simulink model "admire_complete_trim"  (Simulink 3.00)
settings: Solver=ode5  SolverMode=SingleTasking  StartTime=0.0  StopTime=60  FixedStep=0.02  RelTol=1e-3  AbsTol=1e-6
undefined symbols (not defined in the file or in its folder): dalpha_err, dalt_err, dbeta_err, dCl_beta, dCl_dai, dCl_day, dCl_dr, dCl_p, dCl_r, dCm_alpha, dCm_dei, dCm_dey, dCm_dne, dCm_q, dCn_beta, dCn_dna, dCn_dr, dCn_p, dCn_r, dCn_zero, dIxx, dIxz, dIyy, dIzz, dmass, dVt_err, dxcg, dycg, dzcg, u0corr, x00unc
libraries: simulink3 x22, simulink_extras x5
(part 1 of 2)
settings Model: Refine=4  SaveState=on  RTWOptions="-aLogVarNameModifier=\"rt_\" -aExtMode=0 -aRollThreshold=5 -aShowEliminatedStatements=1 -aRTWVerbose=1 -aInlineInvariantSignals=1 -aLocalBlockOutputs=1 -aInlineParameters=0"  RTWTemplateMakefile=grt_adm5p3.tmf  LastModifiedBy=lkh  ModifiedComment=nnt -- Mon Jun 05 13:08:11 2000 -- Version 3.42
settings Model: ModifiedHistory=|
  | nnt -- Mon Jun 05 13:08:11 2000 -- Version 3.42
  | 
  | 
  | nnt -- Mon Jun 05 11:01:33 2000 -- Version 3.41
  | 
  | 
  | nnt -- Mon Jun 05 10:57:40 2000 -- Version 3.40
  | 
  | 
  | nnt -- Mon Jun 05 10:56:46 2000 -- Version 3.39
  | 
  | 
  | hkg -- Thu Apr 13 16:38:30 2000 -- Version 3.38
  | Bug fix: all rate limiters were set with the canard parameters, now they get individual settings..
  | 
  | hkg -- Thu Apr 13 10:24:31 2000 -- Version 3.37
  | Inserted 3.0 version number in Level 1, changed month to April.
  | 
  | hkg -- Tue Apr 11 10:36:55 2000 -- Version 3.36
  | dtz re-connected
  | 
  | hkg -- Tue Apr 11 10:28:52 2000 -- Version 3.35
  | Changed the roll force saturation to +-80 N
  | 
  | hkg -- Tue Apr 11 09:23:02 2000 -- Version 3.34
  | All signal generators on Level 1 are now set to sine wave
  | 
  | hkg -- Mon Apr 10 15:03:16 2000 -- Version 3.33
  | New names for the RL_choice blocks
  | 
  | fosimadmin -- Mon Apr 10 13:44:14 2000 -- Version 3.32
  | Hkg actually. Nothing special
  | 
  | hkg -- Fri Apr 07 14:32:16 2000 -- Version 3.31
  | A few corrections to the names
  | 
  | hkg -- Fri Apr 07 14:16:55 2000 -- Version 3.30
  | Added unique names inside Saab and DASA rate limiters for left elevons, rudder and
  | leading-edge flaps.
  | hkg -- Fri Apr 07 14:04:35 2000 -- Version 3.29
  | Added unique names inside SAAB and DASA rate limiters for canard and right outer and
  | inner elevons.
  | hkg -- Thu Apr 06 17:23:24 2000 -- Version 3.28
  | Inserted unique names for rate limiters and multiport switches in the rate limiter selection blocks.
  | hkg -- Thu Apr 06 16:09:22 2000 -- Version 3.27
  | Disconnected dtz again. Chosen grt_adm5p3.tmf as template makefile. Code generation seems to work.
  | hyd -- Tue Mar 28 15:20:39 2000 -- Version 3.26
  | hyd -- Tue Mar 28 14:28:32 2000 -- Version 3.25
  | hyd -- Tue Mar 28 11:30:24 2000 -- Version 3.24
  | hyd -- Mon Mar 27 15:22:27 2000 -- Version 3.23
  | hyd -- Mon Mar 27 13:42:12 2000 -- Version 3.22
  | hyd -- Mon Mar 27 10:51:54 2000 -- Version 3.21
  | hyd -- Fri Mar 24 13:18:05 2000 -- Version 3.20
  | hyd -- Fri Mar 24 12:50:02 2000 -- Version 3.19
  | hyd -- Fri Mar 24 11:54:23 2000 -- Version 3.18
  | hyd -- Thu Mar 23 15:20:42 2000 -- Version 3.17
  | hyd -- Thu Mar 23 15:17:54 2000 -- Version 3.16
  | hyd -- Wed Mar 22 09:38:49 2000 -- Version 3.15
  | hyd -- Tue Mar 21 14:06:08 2000 -- Version 3.14
  | hyd -- Mon Mar 20 14:42:54 2000 -- Version 3.13
  | hyd -- Wed Mar 15 13:37:48 2000 -- Version 3.12
  | hyd -- Wed Mar 15 12:35:54 2000 -- Version 3.11
  | jnr -- Tue Mar 14 16:36:26 2000 -- Version 3.10
  | jnr -- Tue Mar 14 14:13:39 2000 -- Version 3.9
  | jnr -- Tue Mar 14 14:13:23 2000 -- Version 3.8
  | jnr -- Tue Mar 14 10:09:15 2000 -- Version 3.7
  | jnr -- Tue Mar 14 09:37:34 2000 -- Version 3.6
  | jnr -- Tue Mar 14 09:30:20 2000 -- Version 3.5
  | Add:
  | *proper stick gradients.
  | *correct gains for nz-control according to Åke Hydén.
  | *what transition region between q-control and nz-control is proper??
  | fll -- Fri Mar 03 09:53:48 2000 -- Version 3.4
  | changed name of "dtx" to "dty" (horizontal nozzle deflection)
  | fll -- Thu Mar 02 12:51:23 2000 -- Version 3.3
  | Reducesed the number of integrators to one in the longitudinal controller.
  | fll -- Thu Mar 02 12:30:52 2000 -- Version 3.2
  | Moved the blending function in the Nz and q controller.
  | fll -- Thu Mar 02 10:50:25 2000 -- Version 3.1
  | Changed input blocks to "Signal generator"
  | fll -- Thu Mar 02 10:50:25 2000 -- Version 3.0
  | Version 3.0 is modified according to comments from users

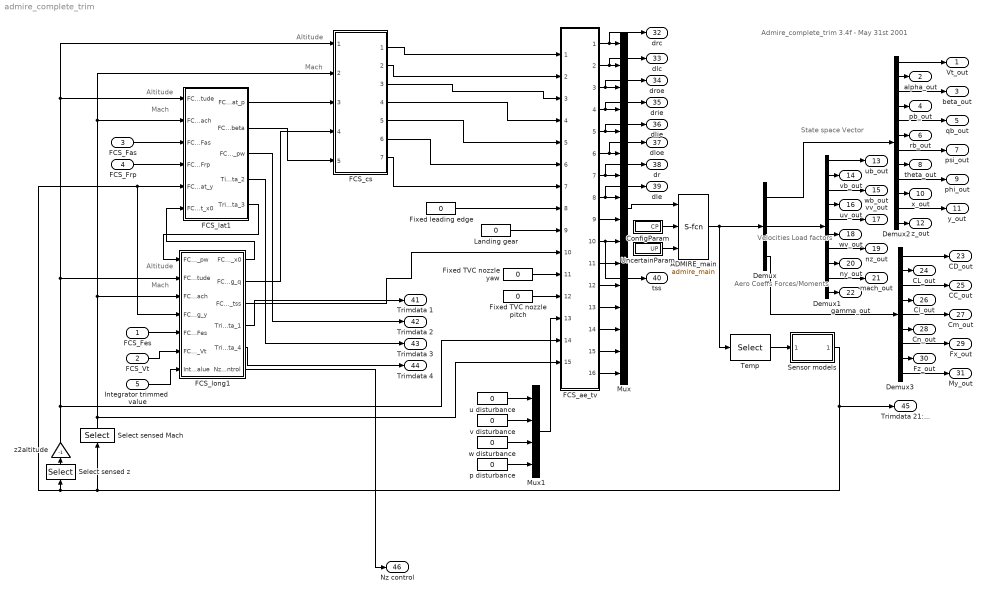
== system admire_complete_trim ==
  note: Admire_complete_trim 3.4f - May 31st 2001
  note: State space Vector
  note: Velocities
      | Load factors
  note: Aero Coeffs
      | Forces/Moments
  note: Altitude
  note: Mach
  note: Mach
  note: Altitude
  note: Altitude
  note: Mach
  FCS_Fes : Inport  Port=1  PortWidth=-1  SampleTime=-1  DataType=auto
      settings: SignalType=auto
  FCS_Vt : Inport  Port=2  PortWidth=-1  SampleTime=-1  DataType=auto
      settings: SignalType=auto
  FCS_Fas : Inport  Port=3  PortWidth=-1  SampleTime=-1  DataType=auto
      settings: SignalType=auto
  FCS_Frp : Inport  Port=4  PortWidth=-1  SampleTime=-1  DataType=auto
      settings: SignalType=auto
  Integrator trimmed  value : Inport  Port=5  PortWidth=-1  SampleTime=-1  DataType=auto
      settings: SignalType=auto
  ADMIRE_main : S-Function  FunctionName=admire_main  Parameters=x0bare zeros(12,1)  PortCounts=[]  SFunctionModules=''
      mask Type: ADMIRE C-code block
      mask Description:
      | Main block describing the ADMIRE.
      | To use HELP, start any Internet browser.
      mask Help:
      | The aircraft it self is a C-code file that calculates the dynamics of the structure and the air surrounding it.<br>
      | The simulation requires an initial vector of values called x0 containing the following variables.<br><br>
      | 
      | Vt_init     --     initial airspeed.                        [m/s]<br>
      | alpha_init --    initial angle of attack.             [rad]<br>
      | beta_init    --   initial angle of sideslip.            [rad]<br>
      | pb_init     --     initial roll angular rate.             [rad/s]<br>
      | qb_init     --     initial pitch angular rate.          [rad/s]<br>
      | rb_init       --    initial yaw angular rate.           [rad/s]<br>
      | psi_init      --    initial euler angles (azimuth)    [rad]<br>
      | theta_init   --   initial (elevation)                      [rad]<br>
      | phi_init      --   initial (bank)                             [rad]<br>
      | xv_init      --    initial x position in Fv                [m]<br>
      | yv_init        --  initial y                                     [m]<br>
      | zv_init       --   initial z                                     [m]<br>
      mask Display:
      | plot([18 12 3 2 2 8 11],[7 4 1 1 2 8 11])
      | plot([13 11 13 15 15 13],[12 11 16 17 13 12])
      | plot([15 17 20 23 30 17],[13 14 24 25 20 14])
      | plot([30 38 40 38 30],[19 31 32 22 19])
      | plot([38.5 41 36 22 41 43 36],[23 21 16 10 8 10 16])
      | plot([15 19 25 24 15],[7 9 9 8 7])
      | plot([8 11 13 14 9 8],[8 11 12 10 7 8])
      | plot([21 23],[9 10])
      | plot([30 31],[20 20.5])
  ConfigParam : Subsystem
  Demux : Demux  Outputs=[12 10 9]
  Demux1 : Demux  Outputs=10
  Demux2 : Demux  Outputs=12
  Demux3 : Demux  Outputs=9
  FCS_ae_tv : Subsystem
      mask Display: disp('Adding\ntrim\nvalues')
  "FCS_cs " : Subsystem
      mask Display: disp('FCS_cs')
  FCS_lat1 : Subsystem
      mask Display: disp('FCS_lat')
  FCS_long1 : Subsystem
      mask Display: disp('FCS_long')
  Fixed TVC nozzle pitch : Constant  Value=0
  Fixed TVC nozzle yaw : Constant  Value=0
  Fixed leading edge : Constant  Value=0
  Landing gear : Constant  Value=0
  Mux : Mux  Inputs=16
      settings: DisplayOption=none
  Mux1 : Mux  Inputs=4
      settings: DisplayOption=none
  Select sensed Mach : Selector  Orientation=up  Elements=21  InputPortWidth=28
  Select sensed z : Selector  Orientation=up  Elements=12  InputPortWidth=28
  Sensor models : Subsystem
      mask Display: disp('Sensors')
  Temp : Selector  Elements=[1:28]  InputPortWidth=31
  UncertainParam : Subsystem
      mask Display: plot([0 10 5 0],[0 0 8.6603 0])
  p disturbance : Constant  Value=0
  u disturbance : Constant  Value=0
  v disturbance : Constant  Value=0
  w disturbance : Constant  Value=0
  z2altitude : Gain  Orientation=up  Gain=-1  SaturateOnIntegerOverflow=off
  Vt_out : Outport  Port=1
  alpha_out : Outport  Port=2
  beta_out : Outport  Port=3
  pb_out : Outport  Port=4
  qb_out : Outport  Port=5
  rb_out : Outport  Port=6
  psi_out : Outport  Port=7
  theta_out : Outport  Port=8
  phi_out : Outport  Port=9
  x_out : Outport  Port=10
  y_out : Outport  Port=11
  z_out : Outport  Port=12
  ub_out : Outport  Port=13
  vb_out : Outport  Port=14
  wb_out : Outport  Port=15
  uv_out : Outport  Port=16
  vv_out : Outport  Port=17
  wv_out : Outport  Port=18
  nz_out : Outport  Port=19
  ny_out : Outport  Port=20
  mach_out : Outport  Port=21
  gamma_out : Outport  Port=22
  CD_out : Outport  Port=23
  CL_out : Outport  Port=24
  CC_out : Outport  Port=25
  Cl_out : Outport  Port=26
  Cm_out : Outport  Port=27
  Cn_out : Outport  Port=28
  Fx_out : Outport  Port=29
  Fz_out : Outport  Port=30
  My_out : Outport  Port=31
  drc : Outport  Port=32
  dlc : Outport  Port=33
  droe : Outport  Port=34
  drie : Outport  Port=35
  dlie : Outport  Port=36
  dloe : Outport  Port=37
  dr : Outport  Port=38
  dle : Outport  Port=39
  tss : Outport  Port=40
  Trimdata 1 : Outport  Port=41
  Trimdata 2 : Outport  Port=42
  Trimdata 3 : Outport  Port=43
  Trimdata 4 : Outport  Port=44
  Trimdata 21:... : Outport  Port=45
  Nz control : Outport  Port=46
  wires:
  FCS_Fes/1 -> FCS_long1/5(FCS_long_Fes)
  FCS_Vt/1 -> FCS_long1/6("FCS_long_Vt ")
  FCS_Fas/1 -> FCS_lat1/3(FCS_lat_Fas)
  FCS_Frp/1 -> FCS_lat1/4(FCS_lat_Frp)
  FCS_lat1/1("FCS_lat_p ") -> "FCS_cs "/3(FCS_cs_p)
  FCS_lat1/2("FCS_lat_beta ") -> "FCS_cs "/5(FCS_cs_beta)
  FCS_lat1/5(Trimdata_3) -> FCS_long1/1("FCS_long_pw ")
  FCS_long1/2(FCS_long_q) -> "FCS_cs "/4(FCS_cs_q)
  FCS_long1/4(Trimdata_1) -> Trimdata 1/1
  FCS_long1/5(Trimdata_4) -> Trimdata 4/1
  FCS_lat1/3(FCS_lat_pw) -> Trimdata 2/1
  FCS_lat1/4(Timdata_2) -> Trimdata 3/1
  FCS_long1/1(FCS_long_x0) -> FCS_lat1/6(FCS_lat_x0)
  Demux/1 -> Demux2/1
  Demux/3 -> Demux3/1
  ADMIRE_main/1 -> Demux/1, Temp/1
  Temp/1 -> Sensor models/1(admire_out)
  Demux3/2 -> CL_out/1
  Demux3/4 -> Cl_out/1
  Demux3/6 -> Cn_out/1
  Demux3/8 -> Fz_out/1
  Demux3/1 -> CD_out/1
  Demux3/3 -> CC_out/1
  Demux3/5 -> Cm_out/1
  Demux3/7 -> Fx_out/1
  Demux3/9 -> My_out/1
  Demux2/2 -> alpha_out/1
  Demux2/4 -> pb_out/1
  Demux2/6 -> rb_out/1
  Demux2/8 -> theta_out/1
  Demux2/10 -> x_out/1
  Demux2/12 -> z_out/1
  Demux2/1 -> Vt_out/1
  Demux2/3 -> beta_out/1
  Demux2/5 -> qb_out/1
  Demux2/7 -> psi_out/1
  Demux2/9 -> phi_out/1
  Demux2/11 -> y_out/1
  Demux/2 -> Demux1/1
  Demux1/2 -> vb_out/1
  Demux1/4 -> uv_out/1
  Demux1/6 -> wv_out/1
  Demux1/8 -> ny_out/1
  Demux1/10 -> gamma_out/1
  Demux1/1 -> ub_out/1
  Demux1/3 -> wb_out/1
  Demux1/5 -> vv_out/1
  Demux1/7 -> nz_out/1
  Demux1/9 -> mach_out/1
  ConfigParam/1(CP) -> ADMIRE_main/2
  UncertainParam/1(UP) -> ADMIRE_main/3
  Mux/1 -> ADMIRE_main/1
  FCS_ae_tv/11(FCS_ae_tv_dty_out) -> Mux/11
  FCS_ae_tv/12("FCS_ae_tv_dtz_out ") -> Mux/12
  FCS_ae_tv/13("FCS_ae_tv_u_dist_out ") -> Mux/13
  FCS_ae_tv/14("FCS_ae_tv_v_dist_out ") -> Mux/14
  FCS_ae_tv/15(FCS_ae_tv_w_dist _out) -> Mux/15
  FCS_ae_tv/16("FCS_ae_tv_p_dist_out ") -> Mux/16
  Fixed TVC nozzle pitch/1 -> FCS_ae_tv/12(FCS_ae_tv_dtz)
  Fixed TVC nozzle yaw/1 -> FCS_ae_tv/11(FCS_ae_tv_dty)
  Landing gear/1 -> FCS_ae_tv/9(FCS_ae_tv_ldg)
  Sensor models/1(admire_sensed_out) -> Trimdata 21:.../1, Select sensed z/1, FCS_long1/4(FCS_long_y), FCS_lat1/5("FCS_lat_y "), Select sensed Mach/1
  "FCS_cs "/1(FCS_cs_drc) -> FCS_ae_tv/1(FCS_ae_tv_drc)
  FCS_ae_tv/1("FCS_ae_tv_drc_out ") -> Mux/1, drc/1
  "FCS_cs "/2(FCS_cs_dlc) -> FCS_ae_tv/2(FCS_ae_tv_dlc)
  FCS_ae_tv/2("FCS_ae_tv_dlc_out ") -> Mux/2, dlc/1
  "FCS_cs "/3(FCS_cs_droe) -> FCS_ae_tv/3(FCS_ae_tv_droe)
  FCS_ae_tv/3("FCS_ae_tv_droe_out ") -> Mux/3, droe/1
  "FCS_cs "/4(FCS_cs_drie) -> FCS_ae_tv/4(FCS_ae_tv_drie)
  FCS_ae_tv/4("FCS_ae_tv_drie_out ") -> Mux/4, drie/1
  "FCS_cs "/5(FCS_cs_dlie) -> FCS_ae_tv/5(FCS_ae_tv_dlie)
  FCS_ae_tv/5("FCS_ae_tv_dlie_out ") -> Mux/5, dlie/1
  "FCS_cs "/6(FCS_cs_dloe) -> FCS_ae_tv/6(FCS_ae_tv_dloe)
  FCS_ae_tv/6("FCS_ae_tv_dloe_out ") -> Mux/6, dloe/1
  "FCS_cs "/7(FCS_cs_dr) -> FCS_ae_tv/7(FCS_ae_tv_dr)
  FCS_ae_tv/7(FCS_ae_tv_dr _out) -> Mux/7, dr/1
  Fixed leading edge/1 -> FCS_ae_tv/8(FCS_ae_tv_dle)
  FCS_ae_tv/8("FCS_ae_tv_dle_out ") -> Mux/8, dle/1
  FCS_long1/3(FCS_long_tss) -> FCS_ae_tv/10(FCS_ae_tv_tss)
  FCS_ae_tv/9(FCS_ae_tv_ldg_out) -> Mux/9
  FCS_ae_tv/10("FCS_ae_tv_tss_out ") -> Mux/10, tss/1
  Integrator trimmed  value/1 -> FCS_long1/7(Integrator value)
  Mux1/1 -> FCS_ae_tv/13(FCS_ae_tv_dist)
  p disturbance/1 -> Mux1/4
  w disturbance/1 -> Mux1/3
  v disturbance/1 -> Mux1/2
  u disturbance/1 -> Mux1/1
  Select sensed z/1 -> z2altitude/1
  Select sensed Mach/1 -> FCS_long1/3(FCS_long_Mach), "FCS_cs "/2(FCS_cs_Mach), FCS_lat1/2("FCS_lat_Mach "), FCS_ae_tv/15(Mach)
  z2altitude/1 -> FCS_long1/2("FCS_long_Altitude "), FCS_lat1/1("FCS_lat_Altitude "), "FCS_cs "/1(FCS_cs_Altitude), FCS_ae_tv/14(Altitude)
  FCS_long1/6(Nz control) -> Nz control/1

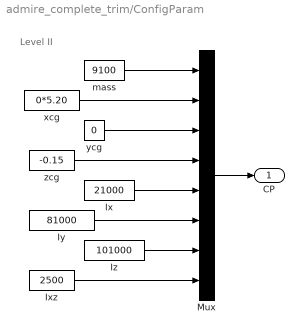
== system admire_complete_trim/ConfigParam ==
  note: Level II
  "Ix " : Constant  Value=21000
  "Ixz " : Constant  Value=2500
  "Iy " : Constant  Value=81000
  "Iz " : Constant  Value=101000
  Mux : Mux  Inputs=8
      settings: DisplayOption=none
  "mass " : Constant  Value=9100
  "xcg " : Constant  Value=0*5.20
  "ycg " : Constant  Value=0
  "zcg " : Constant  Value=-0.15
  CP : Outport  Port=1  InitialOutput=0
  wires:
  "mass "/1 -> Mux/1
  "xcg "/1 -> Mux/2
  "ycg "/1 -> Mux/3
  "zcg "/1 -> Mux/4
  "Ix "/1 -> Mux/5
  "Iy "/1 -> Mux/6
  "Iz "/1 -> Mux/7
  "Ixz "/1 -> Mux/8
  Mux/1 -> CP/1

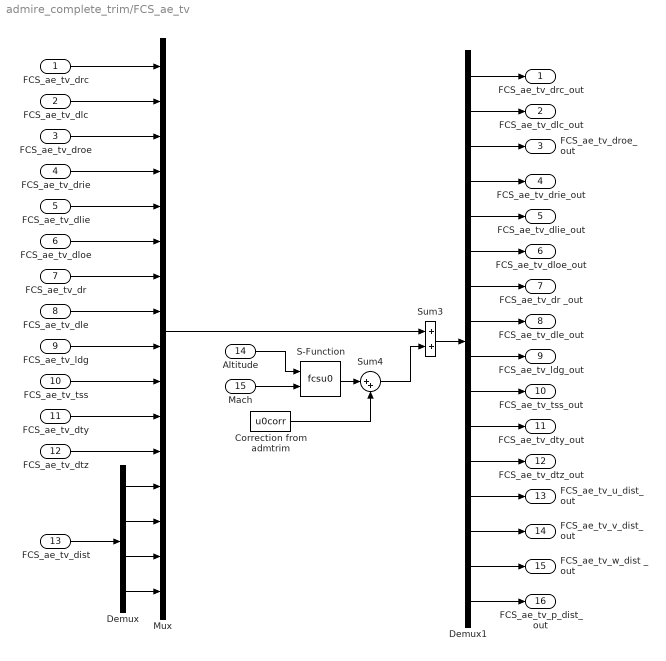
== system admire_complete_trim/FCS_ae_tv ==
  FCS_ae_tv_drc : Inport  Port=1  PortWidth=-1  SampleTime=-1  DataType=auto
      settings: SignalType=auto
  FCS_ae_tv_dlc : Inport  Port=2  PortWidth=-1  SampleTime=-1  DataType=auto
      settings: SignalType=auto
  FCS_ae_tv_droe : Inport  Port=3  PortWidth=-1  SampleTime=-1  DataType=auto
      settings: SignalType=auto
  FCS_ae_tv_drie : Inport  Port=4  PortWidth=-1  SampleTime=-1  DataType=auto
      settings: SignalType=auto
  FCS_ae_tv_dlie : Inport  Port=5  PortWidth=-1  SampleTime=-1  DataType=auto
      settings: SignalType=auto
  FCS_ae_tv_dloe : Inport  Port=6  PortWidth=-1  SampleTime=-1  DataType=auto
      settings: SignalType=auto
  FCS_ae_tv_dr : Inport  Port=7  PortWidth=-1  SampleTime=-1  DataType=auto
      settings: SignalType=auto
  FCS_ae_tv_dle : Inport  Port=8  PortWidth=-1  SampleTime=-1  DataType=auto
      settings: SignalType=auto
  FCS_ae_tv_ldg : Inport  Port=9  PortWidth=-1  SampleTime=-1  DataType=auto
      settings: SignalType=auto
  FCS_ae_tv_tss : Inport  Port=10  PortWidth=-1  SampleTime=-1  DataType=auto
      settings: SignalType=auto
  FCS_ae_tv_dty : Inport  Port=11  PortWidth=-1  SampleTime=-1  DataType=auto
      settings: SignalType=auto
  FCS_ae_tv_dtz : Inport  Port=12  PortWidth=-1  SampleTime=-1  DataType=auto
      settings: SignalType=auto
  FCS_ae_tv_dist : Inport  Port=13  PortWidth=-1  SampleTime=-1  DataType=auto
      settings: SignalType=auto
  Altitude : Inport  Port=14  PortWidth=-1  SampleTime=-1  DataType=auto
      settings: SignalType=auto
  Mach : Inport  Port=15  PortWidth=-1  SampleTime=-1  DataType=auto
      settings: SignalType=auto
  Correction from admtrim : Constant  Value=u0corr
  Demux : Demux  Outputs=4
  Demux1 : Demux  Outputs=16
  Mux : Mux  Inputs=16
  S-Function : S-Function  FunctionName=fcsu0  PortCounts=[]  SFunctionModules=''
  Sum3 : Sum  Inputs=++  SaturateOnIntegerOverflow=on
  Sum4 : Sum  Inputs=|++  SaturateOnIntegerOverflow=on
  "FCS_ae_tv_drc_out " : Outport  Port=1
  "FCS_ae_tv_dlc_out " : Outport  Port=2
  "FCS_ae_tv_droe_out " : Outport  Port=3
  "FCS_ae_tv_drie_out " : Outport  Port=4
  "FCS_ae_tv_dlie_out " : Outport  Port=5
  "FCS_ae_tv_dloe_out " : Outport  Port=6
  FCS_ae_tv_dr _out : Outport  Port=7
  "FCS_ae_tv_dle_out " : Outport  Port=8
  FCS_ae_tv_ldg_out : Outport  Port=9
  "FCS_ae_tv_tss_out " : Outport  Port=10
  FCS_ae_tv_dty_out : Outport  Port=11
  "FCS_ae_tv_dtz_out " : Outport  Port=12
  "FCS_ae_tv_u_dist_out " : Outport  Port=13
  "FCS_ae_tv_v_dist_out " : Outport  Port=14
  FCS_ae_tv_w_dist _out : Outport  Port=15
  "FCS_ae_tv_p_dist_out " : Outport  Port=16
  wires:
  FCS_ae_tv_dist/1 -> Demux/1
  FCS_ae_tv_drc/1 -> Mux/1
  FCS_ae_tv_dlc/1 -> Mux/2
  FCS_ae_tv_droe/1 -> Mux/3
  FCS_ae_tv_drie/1 -> Mux/4
  FCS_ae_tv_dlie/1 -> Mux/5
  FCS_ae_tv_dloe/1 -> Mux/6
  FCS_ae_tv_dr/1 -> Mux/7
  FCS_ae_tv_dle/1 -> Mux/8
  FCS_ae_tv_dty/1 -> Mux/11
  FCS_ae_tv_dtz/1 -> Mux/12
  Demux/1 -> Mux/13
  Demux/2 -> Mux/14
  Demux/3 -> Mux/15
  Demux/4 -> Mux/16
  FCS_ae_tv_ldg/1 -> Mux/9
  FCS_ae_tv_tss/1 -> Mux/10
  Sum3/1 -> Demux1/1
  Demux1/3 -> "FCS_ae_tv_droe_out "/1
  Demux1/4 -> "FCS_ae_tv_drie_out "/1
  Demux1/5 -> "FCS_ae_tv_dlie_out "/1
  Demux1/6 -> "FCS_ae_tv_dloe_out "/1
  Demux1/7 -> FCS_ae_tv_dr _out/1
  Demux1/8 -> "FCS_ae_tv_dle_out "/1
  Demux1/11 -> FCS_ae_tv_dty_out/1
  Demux1/12 -> "FCS_ae_tv_dtz_out "/1
  Demux1/13 -> "FCS_ae_tv_u_dist_out "/1
  Demux1/14 -> "FCS_ae_tv_v_dist_out "/1
  Demux1/15 -> FCS_ae_tv_w_dist _out/1
  Demux1/16 -> "FCS_ae_tv_p_dist_out "/1
  Demux1/2 -> "FCS_ae_tv_dlc_out "/1
  Demux1/1 -> "FCS_ae_tv_drc_out "/1
  Mux/1 -> Sum3/1
  S-Function/1 -> Sum4/1
  Correction from admtrim/1 -> Sum4/2
  Demux1/9 -> FCS_ae_tv_ldg_out/1
  Demux1/10 -> "FCS_ae_tv_tss_out "/1
  Altitude/1 -> S-Function/1
  Mach/1 -> S-Function/2
  Sum4/1 -> Sum3/2

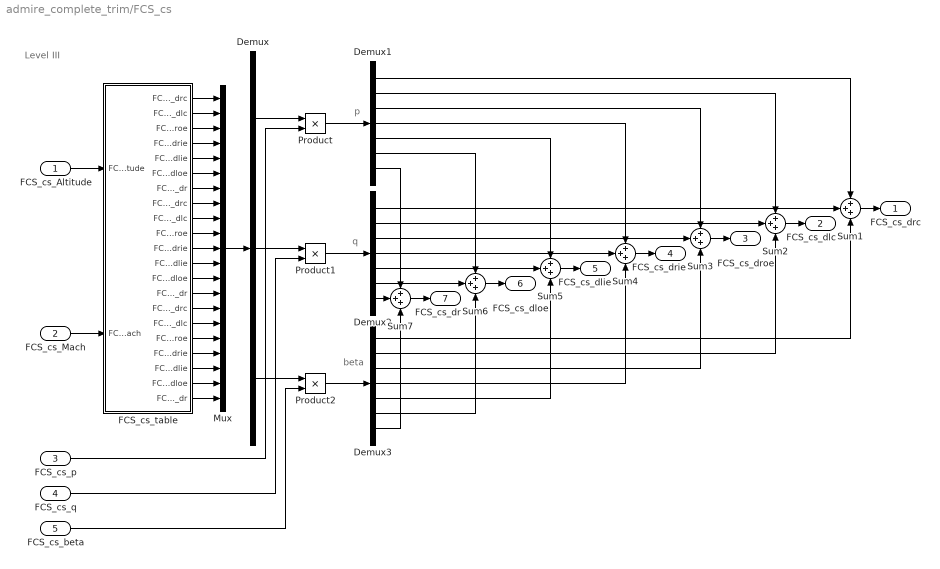
== system admire_complete_trim/FCS_cs  ==
  note: Level III
  note: beta
  note: q
  note: p
  FCS_cs_Altitude : Inport  Port=1  PortWidth=-1  SampleTime=-1  DataType=auto
      settings: SignalType=auto
  FCS_cs_Mach : Inport  Port=2  PortWidth=-1  SampleTime=-1  DataType=auto
      settings: SignalType=auto
  FCS_cs_p : Inport  Port=3  PortWidth=-1  SampleTime=-1  DataType=auto
      settings: SignalType=auto
  FCS_cs_q : Inport  Port=4  PortWidth=-1  SampleTime=-1  DataType=auto
      settings: SignalType=auto
  FCS_cs_beta : Inport  Port=5  PortWidth=-1  SampleTime=-1  DataType=auto
      settings: SignalType=auto
  Demux : Demux  Outputs=[7 7 7]
  Demux1 : Demux  Outputs=7
  Demux2 : Demux  Outputs=7
  Demux3 : Demux  Outputs=7
  FCS_cs_table : Subsystem
      mask Display: disp('FCS_cs_table')
  Mux : Mux  Inputs=21
  Product : Product  Inputs=2  SaturateOnIntegerOverflow=on
  Product1 : Product  Inputs=2  SaturateOnIntegerOverflow=on
  Product2 : Product  Inputs=2  SaturateOnIntegerOverflow=on
  Sum{1..7} (7 alike) : Sum  Inputs=3  SaturateOnIntegerOverflow=on
  FCS_cs_drc : Outport  Port=1
  FCS_cs_dlc : Outport  Port=2
  FCS_cs_droe : Outport  Port=3
  FCS_cs_drie : Outport  Port=4
  FCS_cs_dlie : Outport  Port=5
  FCS_cs_dloe : Outport  Port=6
  FCS_cs_dr : Outport  Port=7
  wires:
  Sum1/1 -> FCS_cs_drc/1
  Demux3/1 -> Sum1/3
  Demux1/1 -> Sum1/1
  Sum2/1 -> FCS_cs_dlc/1
  Demux3/2 -> Sum2/3
  Demux1/2 -> Sum2/1
  Demux2/1 -> Sum1/2
  Sum3/1 -> FCS_cs_droe/1
  Demux3/3 -> Sum3/3
  Demux1/3 -> Sum3/1
  Demux2/2 -> Sum2/2
  Sum4/1 -> FCS_cs_drie/1
  Demux3/4 -> Sum4/3
  Demux1/4 -> Sum4/1
  Demux2/3 -> Sum3/2
  Sum5/1 -> FCS_cs_dlie/1
  Demux3/5 -> Sum5/3
  Demux1/5 -> Sum5/1
  Demux2/4 -> Sum4/2
  Sum6/1 -> FCS_cs_dloe/1
  Demux3/6 -> Sum6/3
  Demux1/6 -> Sum6/1
  Demux2/5 -> Sum5/2
  Sum7/1 -> FCS_cs_dr/1
  Demux3/7 -> Sum7/3
  Demux1/7 -> Sum7/1
  Demux2/7 -> Sum7/2
  Demux2/6 -> Sum6/2
  Product2/1 -> Demux3/1
  Product1/1 -> Demux2/1
  Product/1 -> Demux1/1
  FCS_cs_table/21(FCS_cs_table_beta_dr) -> Mux/21
  FCS_cs_table/20(FCS_cs_table_beta_dloe) -> Mux/20
  FCS_cs_table/19(FCS_cs_table_beta_dlie) -> Mux/19
  FCS_cs_table/18(FCS_cs_table_beta_drie) -> Mux/18
  FCS_cs_table/17(FCS_cs_table_beta_droe) -> Mux/17
  FCS_cs_table/16(FCS_cs_table_beta_dlc) -> Mux/16
  FCS_cs_table/15(FCS_cs_table_beta_drc) -> Mux/15
  FCS_cs_table/13(FCS_cs_table_q_dloe) -> Mux/13
  FCS_cs_table/14(FCS_cs_table_q_dr) -> Mux/14
  FCS_cs_table/12(FCS_cs_table_q_dlie) -> Mux/12
  FCS_cs_table/11(FCS_cs_table_q_drie) -> Mux/11
  FCS_cs_table/10(FCS_cs_table_q_droe) -> Mux/10
  FCS_cs_table/9(FCS_cs_table_q_dlc) -> Mux/9
  FCS_cs_table/8(FCS_cs_table_q_drc) -> Mux/8
  FCS_cs_table/7(FCS_cs_table_p_dr) -> Mux/7
  FCS_cs_table/6(FCS_cs_table_p_dloe) -> Mux/6
  FCS_cs_table/5(FCS_cs_table_p_dlie) -> Mux/5
  FCS_cs_table/4(FCS_cs_table_p_drie) -> Mux/4
  FCS_cs_table/3(FCS_cs_table_p_droe) -> Mux/3
  FCS_cs_table/2(FCS_cs_table_p_dlc) -> Mux/2
  FCS_cs_table/1(FCS_cs_table_p_drc) -> Mux/1
  FCS_cs_Mach/1 -> FCS_cs_table/2(FCS_cs_table_Mach)
  FCS_cs_Altitude/1 -> FCS_cs_table/1(FCS_cs_table_Altitude)
  FCS_cs_beta/1 -> Product2/2
  FCS_cs_q/1 -> Product1/2
  FCS_cs_p/1 -> Product/2
  Demux/3 -> Product2/1
  Demux/2 -> Product1/1
  Demux/1 -> Product/1
  Mux/1 -> Demux/1

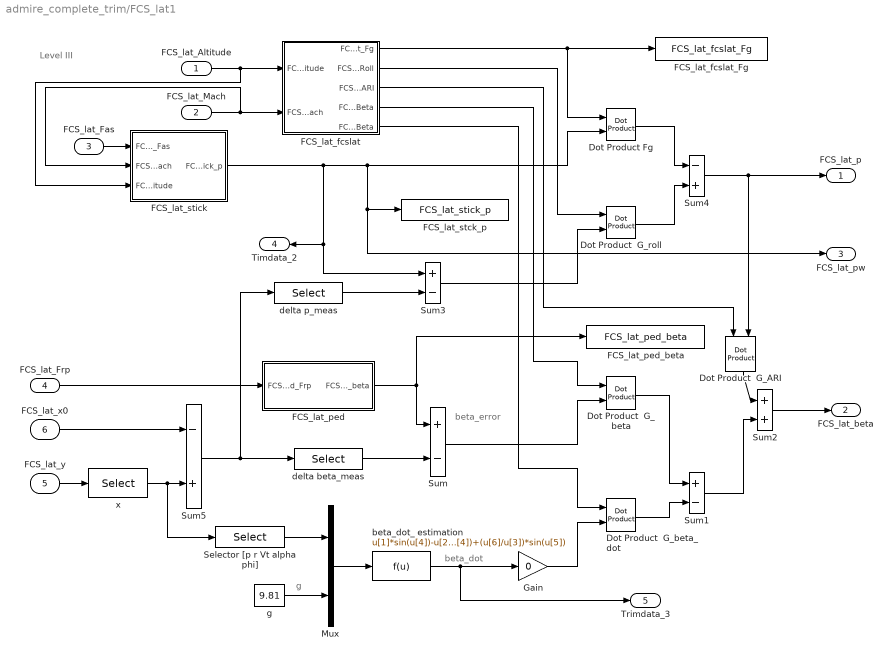
== system admire_complete_trim/FCS_lat1 ==
  note: g
  note: beta_dot
  note: beta_error
  note: Level III
  "FCS_lat_Altitude " : Inport  Port=1  PortWidth=-1  SampleTime=-1  DataType=auto
      settings: SignalType=auto
  "FCS_lat_Mach " : Inport  Port=2  PortWidth=-1  SampleTime=-1  DataType=auto
      settings: SignalType=auto
  FCS_lat_Fas : Inport  Port=3  PortWidth=-1  SampleTime=-1  DataType=auto
      settings: SignalType=auto
  FCS_lat_Frp : Inport  Port=4  PortWidth=-1  SampleTime=-1  DataType=auto
      settings: SignalType=auto
  "FCS_lat_y " : Inport  Port=5  PortWidth=-1  SampleTime=-1  DataType=auto
      settings: SignalType=auto
  FCS_lat_x0 : Inport  Port=6  PortWidth=-1  SampleTime=-1  DataType=auto
      settings: SignalType=auto
  "  x" : Selector  Elements=[1:12]  InputPortWidth=28
  Dot Product Fg : simulink3/Math/Dot Product
  Dot Product  G_ARI : simulink3/Math/Dot Product  Orientation=down
  Dot Product  G_beta : simulink3/Math/Dot Product
  Dot Product  G_beta_dot : simulink3/Math/Dot Product
  Dot Product  G_roll : simulink3/Math/Dot Product
  FCS_lat_fcslat : Subsystem
      mask Display: disp('Calc of lateral\namplfication\n factors')
  FCS_lat_fcslat_Fg : ToWorkspace  VariableName=FCS_lat_fcslat_Fg  SampleTime=-1  SaveFormat=Matrix
  FCS_lat_ped : Subsystem
      mask Display: disp('FCS lateral pedal\nforce N to beta rad')
  FCS_lat_ped_beta : ToWorkspace  VariableName=FCS_lat_ped_beta  SampleTime=-1  SaveFormat=Matrix
  FCS_lat_stck_p : ToWorkspace  VariableName=FCS_lat_stick_p  SampleTime=-1  SaveFormat=Matrix
  FCS_lat_stick : Subsystem
      mask Display: disp('FCS lateral stick\ngradient\n N to rad/s')
  Gain : Gain  Gain=0  SaturateOnIntegerOverflow=on
  Mux : Mux  Inputs=2
      settings: DisplayOption=none
  Selector [p r Vt alpha phi] : Selector  Elements=[4 6 1 2 9]  InputPortWidth=12
  Sum : Sum  Inputs=+-  SaturateOnIntegerOverflow=on
  Sum1 : Sum  Inputs=+-  SaturateOnIntegerOverflow=on
  Sum2 : Sum  Inputs=++  SaturateOnIntegerOverflow=on
  Sum3 : Sum  Inputs=+-  SaturateOnIntegerOverflow=on
  Sum4 : Sum  Inputs=-+  SaturateOnIntegerOverflow=on
  Sum5 : Sum  Inputs=-+  SaturateOnIntegerOverflow=on
  beta_dot_ estimation : Fcn  Expr=u[1]*sin(u[4])-u[2]*cos(u[4])+(u[6]/u[3])*sin(u[5])
  delta beta_meas : Selector  Elements=3  InputPortWidth=12
  delta p_meas : Selector  Elements=4  InputPortWidth=12
  g : Constant  Value=9.81
  "FCS_lat_p " : Outport  Port=1  InitialOutput=0
  "FCS_lat_beta " : Outport  Port=2  InitialOutput=0
  FCS_lat_pw : Outport  Port=3  InitialOutput=0
  Timdata_2 : Outport  Orientation=left  Port=4  InitialOutput=0
  Trimdata_3 : Outport  Port=5  InitialOutput=0
  wires:
  FCS_lat_Fas/1 -> FCS_lat_stick/1("FCS_lat_stick_Fas ")
  delta p_meas/1 -> Sum3/2
  Mux/1 -> beta_dot_ estimation/1
  Selector [p r Vt alpha phi]/1 -> Mux/1
  g/1 -> Mux/2
  Sum3/1 -> Dot Product  G_roll/2
  Dot Product  G_roll/1 -> Sum4/2
  Dot Product Fg/1 -> Sum4/1
  Dot Product  G_beta/1 -> Sum1/1
  Dot Product  G_beta_dot/1 -> Sum1/2
  Sum4/1 -> Dot Product  G_ARI/2, "FCS_lat_p "/1
  Dot Product  G_ARI/1 -> Sum2/1
  Sum2/1 -> "FCS_lat_beta "/1
  Sum1/1 -> Sum2/2
  FCS_lat_stick/1(FCS_lat_stick_p) -> Dot Product Fg/2, FCS_lat_pw/1, FCS_lat_stck_p/1, Sum3/1, Timdata_2/1
  FCS_lat_fcslat/2(FCS_lat_fcslat_GRoll) -> Dot Product  G_roll/1
  FCS_lat_fcslat/3(FCS_lat_fcslat_GARI) -> Dot Product  G_ARI/1
  FCS_lat_fcslat/4(FCS_lat_fcslat_GBeta) -> Dot Product  G_beta/1
  FCS_lat_fcslat/5(FCS_lat_fcslat_dGBeta) -> Dot Product  G_beta_dot/1
  delta beta_meas/1 -> Sum/2
  Sum/1 -> Dot Product  G_beta/2
  FCS_lat_Frp/1 -> FCS_lat_ped/1(FCS_lat_ped_Frp)
  FCS_lat_ped/1(FCS_lat_ped_beta) -> Sum/1, FCS_lat_ped_beta/1
  "FCS_lat_Altitude "/1 -> FCS_lat_fcslat/1(FCS_lat_fcslat_Altitude), FCS_lat_stick/3("FCS_lat_stick_Altitude ")
  "FCS_lat_Mach "/1 -> FCS_lat_stick/2("FCS_lat_stick_Mach "), FCS_lat_fcslat/2(FCS_lat_fcslat_Mach)
  "FCS_lat_y "/1 -> "  x"/1
  FCS_lat_x0/1 -> Sum5/1
  "  x"/1 -> Sum5/2, Selector [p r Vt alpha phi]/1
  Sum5/1 -> delta beta_meas/1, delta p_meas/1
  FCS_lat_fcslat/1(FCS_lat_fcslat_Fg) -> Dot Product Fg/1, FCS_lat_fcslat_Fg/1
  Gain/1 -> Dot Product  G_beta_dot/2
  beta_dot_ estimation/1 -> Gain/1, Trimdata_3/1

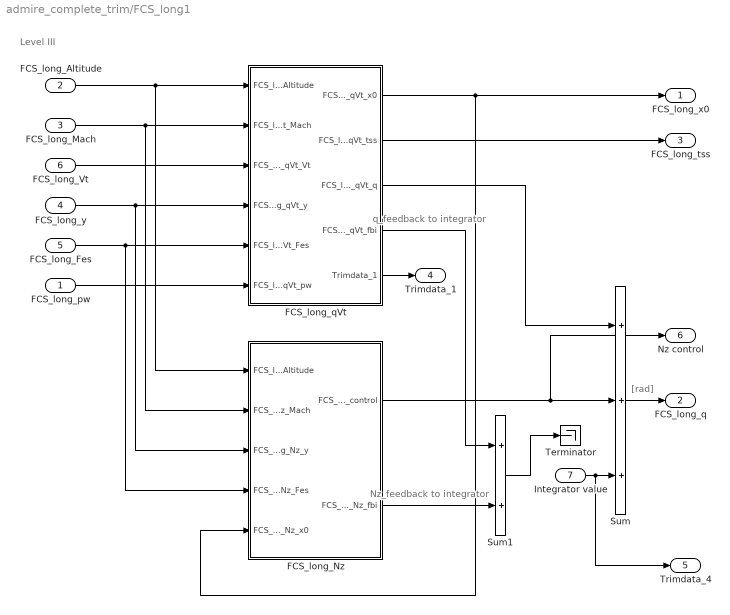
== system admire_complete_trim/FCS_long1 ==
  note: Level III
  note: q_feedback
      | to integrator
  note: Nz_feedback
      | to integrator
  note: [rad]
  "FCS_long_pw " : Inport  Port=1  PortWidth=-1  SampleTime=-1  DataType=auto
      settings: SignalType=auto
  "FCS_long_Altitude " : Inport  Port=2  PortWidth=-1  SampleTime=-1  DataType=auto
      settings: SignalType=auto
  FCS_long_Mach : Inport  Port=3  PortWidth=-1  SampleTime=-1  DataType=auto
      settings: SignalType=auto
  FCS_long_y : Inport  Port=4  PortWidth=-1  SampleTime=-1  DataType=auto
      settings: SignalType=auto
  FCS_long_Fes : Inport  Port=5  PortWidth=-1  SampleTime=-1  DataType=auto
      settings: SignalType=auto
  "FCS_long_Vt " : Inport  Port=6  PortWidth=-1  SampleTime=-1  DataType=auto
      settings: SignalType=auto
  Integrator value : Inport  Port=7  PortWidth=-1  SampleTime=-1  DataType=auto
      settings: SignalType=auto
  FCS_long_Nz : Subsystem
      mask Display: disp('FCS_long_Nz')
  FCS_long_qVt : Subsystem
      mask Display: disp('FCS_long_qVt')
  Sum : Sum  Inputs=+++  SaturateOnIntegerOverflow=on
  Sum1 : Sum  Inputs=++  SaturateOnIntegerOverflow=on
  Terminator : Terminator
  FCS_long_x0 : Outport  Port=1  InitialOutput=0
  FCS_long_q : Outport  Port=2  InitialOutput=0
  FCS_long_tss : Outport  Port=3  InitialOutput=0
  Trimdata_1 : Outport  Port=4  InitialOutput=0
  Trimdata_4 : Outport  Port=5  InitialOutput=0
  Nz control : Outport  Port=6  InitialOutput=0
  wires:
  "FCS_long_Vt "/1 -> FCS_long_qVt/3(FCS_long_qVt_Vt)
  FCS_long_Mach/1 -> FCS_long_qVt/2(FCS_long_qVt_Mach), FCS_long_Nz/2("FCS_long_Nz_Mach ")
  FCS_long_y/1 -> FCS_long_qVt/4(FCS_long_qVt_y), FCS_long_Nz/3(FCS_long_Nz_y)
  FCS_long_qVt/1(FCS_long_qVt_x0) -> FCS_long_x0/1, FCS_long_Nz/5(FCS_long_Nz_x0)
  FCS_long_Fes/1 -> FCS_long_qVt/5(FCS_long_qVt_Fes), FCS_long_Nz/4(FCS_long_Nz_Fes)
  "FCS_long_pw "/1 -> FCS_long_qVt/6("FCS_long_qVt_pw ")
  FCS_long_qVt/2(FCS_long_qVt_tss) -> FCS_long_tss/1
  FCS_long_qVt/3(FCS_long_qVt_q) -> Sum/1
  FCS_long_qVt/4(FCS_long_qVt_fbi) -> Sum1/1
  FCS_long_Nz/2(FCS_long_Nz_fbi) -> Sum1/2
  "FCS_long_Altitude "/1 -> FCS_long_qVt/1(FCS_long_qVt_Altitude), FCS_long_Nz/1("FCS_long_Nz_Altitude ")
  Sum/1 -> FCS_long_q/1
  FCS_long_qVt/5(Trimdata_1) -> Trimdata_1/1
  Integrator value/1 -> Sum/3, Trimdata_4/1
  Sum1/1 -> Terminator/1
  FCS_long_Nz/1(FCS_long_Nz_control) -> Sum/2, Nz control/1

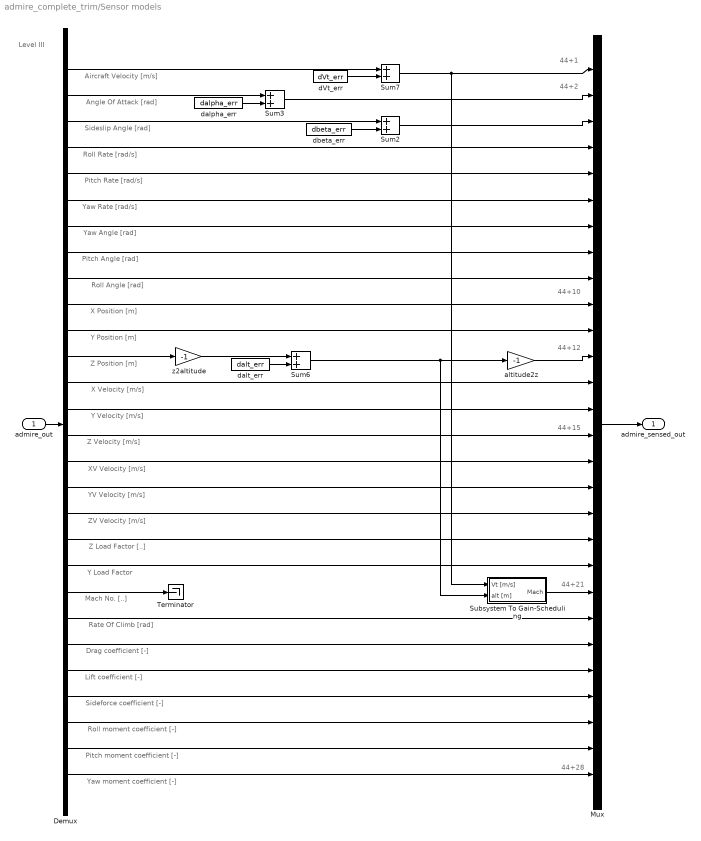
== system admire_complete_trim/Sensor models ==
  note: Aircraft Velocity [m/s]
  note: Angle Of Attack [rad]
  note: Sideslip Angle [rad]
  note: Roll Rate [rad/s]
  note: Pitch Rate [rad/s]
  note: Yaw Rate [rad/s]
  note: Yaw Angle [rad]
  note: Pitch Angle [rad]
  note: Roll Angle [rad]
  note: X Position [m]
  note: Y Position [m]
  note: Z Position [m]
  note: X Velocity [m/s]
  note: Y Velocity [m/s]
  note: Z Velocity [m/s]
  note: ZV Velocity [m/s]
  note: YV Velocity [m/s]
  note: XV Velocity [m/s]
  note: Z Load Factor [..]
  note: Y Load Factor
  note: Mach No. [..]
  note: Rate Of Climb [rad]
  note: Drag coefficient [-]
  note: Lift coefficient [-]
  note: Sideforce coefficient [-]
  note: Roll moment coefficient [-]
  note: Pitch moment coefficient [-]
  note: Yaw moment coefficient [-]
  note: Level III
  note: 44+1
  note: 44+2
  note: 44+10
  note: 44+15
  note: 44+21
  note: 44+28
  note: 44+12
  admire_out : Inport  Port=1  PortWidth=-1  SampleTime=-1  DataType=auto
      settings: SignalType=auto
  Demux : Demux  Outputs=28
  Mux : Mux  Inputs=28
      settings: DisplayOption=none
  Subsystem To Gain-Scheduling : Subsystem
  Sum{2..3,6..7} (4 alike) : Sum  Inputs=++  SaturateOnIntegerOverflow=on
  Terminator : Terminator
  altitude2z : Gain  Gain=-1  SaturateOnIntegerOverflow=off
  dVt_err : Constant  Value=dVt_err
  dalpha_err : Constant  Value=dalpha_err
  dalt_err : Constant  Value=dalt_err
  dbeta_err : Constant  Value=dbeta_err
  z2altitude : Gain  Gain=-1  SaturateOnIntegerOverflow=off
  admire_sensed_out : Outport  Port=1
  wires:
  Demux/24 -> Mux/24
  Demux/25 -> Mux/25
  Demux/26 -> Mux/26
  Demux/27 -> Mux/27
  Demux/28 -> Mux/28
  admire_out/1 -> Demux/1
  Demux/11 -> Mux/11
  Demux/13 -> Mux/13
  Demux/14 -> Mux/14
  Demux/15 -> Mux/15
  Demux/16 -> Mux/16
  Demux/17 -> Mux/17
  Demux/18 -> Mux/18
  Demux/20 -> Mux/20
  Demux/22 -> Mux/22
  Demux/23 -> Mux/23
  Demux/21 -> Terminator/1
  Mux/1 -> admire_sensed_out/1
  Subsystem To Gain-Scheduling/1(Mach) -> Mux/21
  Demux/7 -> Mux/7
  dalt_err/1 -> Sum6/2
  Demux/12 -> z2altitude/1
  z2altitude/1 -> Sum6/1
  Demux/10 -> Mux/10
  Sum7/1 -> Mux/1, Subsystem To Gain-Scheduling/1(Vt [m/s])
  Sum2/1 -> Mux/3
  Demux/4 -> Mux/4
  Demux/5 -> Mux/5
  Demux/6 -> Mux/6
  Demux/8 -> Mux/8
  Demux/9 -> Mux/9
  Demux/19 -> Mux/19
  dalpha_err/1 -> Sum3/2
  Demux/2 -> Sum3/1
  dbeta_err/1 -> Sum2/2
  Demux/3 -> Sum2/1
  Sum3/1 -> Mux/2
  dVt_err/1 -> Sum7/2
  Demux/1 -> Sum7/1
  Sum6/1 -> Subsystem To Gain-Scheduling/2(alt [m]), altitude2z/1
  altitude2z/1 -> Mux/12

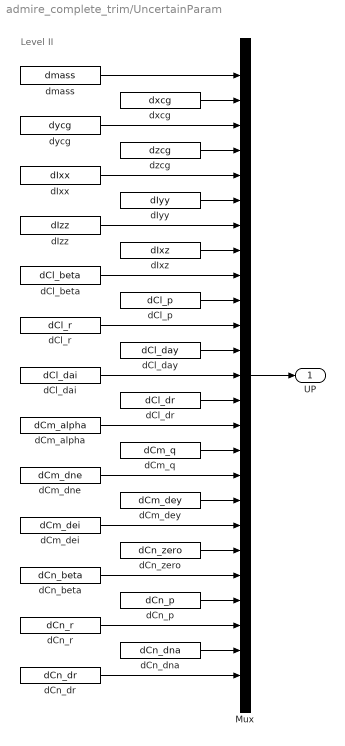
== system admire_complete_trim/UncertainParam ==
  note: Level II
  Mux : Mux  Inputs=25
      settings: DisplayOption=none
  "dCl_beta " : Constant  Value=dCl_beta
  "dCl_dai " : Constant  Value=dCl_dai
  dCl_day : Constant  Value=dCl_day
  "dCl_dr " : Constant  Value=dCl_dr
  "dCl_p " : Constant  Value=dCl_p
  "dCl_r " : Constant  Value=dCl_r
  "dCm_alpha " : Constant  Value=dCm_alpha
  "dCm_dei " : Constant  Value=dCm_dei
  "dCm_dey " : Constant  Value=dCm_dey
  "dCm_dne " : Constant  Value=dCm_dne
  "dCm_q " : Constant  Value=dCm_q
  "dCn_beta " : Constant  Value=dCn_beta
  dCn_dna : Constant  Value=dCn_dna
  "dCn_dr " : Constant  Value=dCn_dr
  "dCn_p " : Constant  Value=dCn_p
  "dCn_r " : Constant  Value=dCn_r
  dCn_zero : Constant  Value=dCn_zero
  dIxx : Constant  Value=dIxx
  dIxz : Constant  Value=dIxz
  "dIyy " : Constant  Value=dIyy
  "dIzz " : Constant  Value=dIzz
  "dmass " : Constant  Value=dmass
  dxcg : Constant  Value=dxcg
  "dycg " : Constant  Value=dycg
  "dzcg " : Constant  Value=dzcg
  UP : Outport  Port=1  InitialOutput=0
  wires:
  dCn_dna/1 -> Mux/24
  "dmass "/1 -> Mux/1
  "dycg "/1 -> Mux/3
  dxcg/1 -> Mux/2
  "dzcg "/1 -> Mux/4
  dIxx/1 -> Mux/5
  "dIyy "/1 -> Mux/6
  "dIzz "/1 -> Mux/7
  dIxz/1 -> Mux/8
  "dCl_beta "/1 -> Mux/9
  "dCl_p "/1 -> Mux/10
  "dCl_r "/1 -> Mux/11
  dCl_day/1 -> Mux/12
  "dCl_dai "/1 -> Mux/13
  "dCl_dr "/1 -> Mux/14
  "dCm_alpha "/1 -> Mux/15
  "dCm_q "/1 -> Mux/16
  "dCm_dey "/1 -> Mux/18
  dCn_zero/1 -> Mux/20
  "dCn_p "/1 -> Mux/22
  Mux/1 -> UP/1
  "dCm_dne "/1 -> Mux/17
  "dCm_dei "/1 -> Mux/19
  "dCn_beta "/1 -> Mux/21
  "dCn_dr "/1 -> Mux/25
  "dCn_r "/1 -> Mux/23

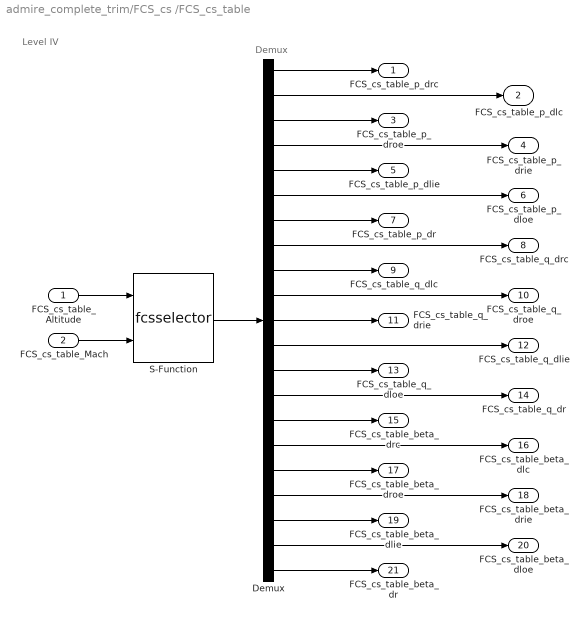
== system admire_complete_trim/FCS_cs /FCS_cs_table ==
  note: Demux
  note: Level IV
  FCS_cs_table_Altitude : Inport  Port=1  PortWidth=-1  SampleTime=-1  DataType=auto
      settings: SignalType=auto
  FCS_cs_table_Mach : Inport  Port=2  PortWidth=-1  SampleTime=-1  DataType=auto
      settings: SignalType=auto
  Demux : Demux  Outputs=21
  S-Function : S-Function  FunctionName=fcsselector  PortCounts=[]  SFunctionModules=''
  FCS_cs_table_p_drc : Outport  Port=1
  FCS_cs_table_p_dlc : Outport  Port=2
  FCS_cs_table_p_droe : Outport  Port=3
  FCS_cs_table_p_drie : Outport  Port=4
  FCS_cs_table_p_dlie : Outport  Port=5
  FCS_cs_table_p_dloe : Outport  Port=6
  FCS_cs_table_p_dr : Outport  Port=7
  FCS_cs_table_q_drc : Outport  Port=8
  FCS_cs_table_q_dlc : Outport  Port=9
  FCS_cs_table_q_droe : Outport  Port=10
  FCS_cs_table_q_drie : Outport  Port=11
  FCS_cs_table_q_dlie : Outport  Port=12
  FCS_cs_table_q_dloe : Outport  Port=13
  FCS_cs_table_q_dr : Outport  Port=14
  FCS_cs_table_beta_drc : Outport  Port=15
  FCS_cs_table_beta_dlc : Outport  Port=16
  FCS_cs_table_beta_droe : Outport  Port=17
  FCS_cs_table_beta_drie : Outport  Port=18
  FCS_cs_table_beta_dlie : Outport  Port=19
  FCS_cs_table_beta_dloe : Outport  Port=20
  FCS_cs_table_beta_dr : Outport  Port=21
  wires:
  Demux/1 -> FCS_cs_table_p_drc/1
  Demux/14 -> FCS_cs_table_q_dr/1
  Demux/20 -> FCS_cs_table_beta_dloe/1
  Demux/18 -> FCS_cs_table_beta_drie/1
  Demux/16 -> FCS_cs_table_beta_dlc/1
  Demux/12 -> FCS_cs_table_q_dlie/1
  Demux/10 -> FCS_cs_table_q_droe/1
  Demux/8 -> FCS_cs_table_q_drc/1
  Demux/6 -> FCS_cs_table_p_dloe/1
  Demux/4 -> FCS_cs_table_p_drie/1
  Demux/2 -> FCS_cs_table_p_dlc/1
  Demux/21 -> FCS_cs_table_beta_dr/1
  Demux/19 -> FCS_cs_table_beta_dlie/1
  Demux/17 -> FCS_cs_table_beta_droe/1
  Demux/15 -> FCS_cs_table_beta_drc/1
  Demux/13 -> FCS_cs_table_q_dloe/1
  Demux/11 -> FCS_cs_table_q_drie/1
  Demux/9 -> FCS_cs_table_q_dlc/1
  Demux/7 -> FCS_cs_table_p_dr/1
  Demux/5 -> FCS_cs_table_p_dlie/1
  Demux/3 -> FCS_cs_table_p_droe/1
  S-Function/1 -> Demux/1
  FCS_cs_table_Mach/1 -> S-Function/2
  FCS_cs_table_Altitude/1 -> S-Function/1

== system admire_complete_trim/FCS_lat1/FCS_lat_fcslat ==
  note: Level IV
  note: S-function
  FCS_lat_fcslat_Altitude : Inport  Port=1  PortWidth=-1  SampleTime=-1  DataType=auto
      settings: SignalType=auto
  FCS_lat_fcslat_Mach : Inport  Port=2  PortWidth=-1  SampleTime=-1  DataType=auto
      settings: SignalType=auto
  S-Function : S-Function  FunctionName=fcslateral  PortCounts=[]  SFunctionModules=''
  FCS_lat_fcslat_Fg : Outport  Port=1
  FCS_lat_fcslat_GRoll : Outport  Port=2
  FCS_lat_fcslat_GARI : Outport  Port=3
  FCS_lat_fcslat_GBeta : Outport  Port=4
  FCS_lat_fcslat_dGBeta : Outport  Port=5
  wires:
  FCS_lat_fcslat_Altitude/1 -> S-Function/1
  FCS_lat_fcslat_Mach/1 -> S-Function/2
  S-Function/1 -> FCS_lat_fcslat_Fg/1
  S-Function/2 -> FCS_lat_fcslat_GBeta/1
  S-Function/3 -> FCS_lat_fcslat_dGBeta/1
  S-Function/4 -> FCS_lat_fcslat_GARI/1
  S-Function/5 -> FCS_lat_fcslat_GRoll/1

== system admire_complete_trim/FCS_lat1/FCS_lat_ped ==
  note: Level IV
  FCS_lat_ped_Frp : Inport  Port=1  PortWidth=-1  SampleTime=-1  DataType=auto
      settings: SignalType=auto
  Degrees to Radians : simulink_extras/Transformations/Degrees to Radians
  Look-Up Table Frp gradient : Lookup  InputValues=[-200 0 200]  OutputValues=[5 0 -5]
  Saturation : Saturate  UpperLimit=200  LowerLimit=-200
  FCS_lat_ped_beta : Outport  Port=1
  wires:
  Saturation/1 -> Look-Up Table Frp gradient/1
  FCS_lat_ped_Frp/1 -> Saturation/1
  Degrees to Radians/1 -> FCS_lat_ped_beta/1
  Look-Up Table Frp gradient/1 -> Degrees to Radians/1

== system admire_complete_trim/FCS_lat1/FCS_lat_stick ==
  note: Level IV
  "FCS_lat_stick_Fas " : Inport  Port=1  PortWidth=-1  SampleTime=-1  DataType=auto
      settings: SignalType=auto
  "FCS_lat_stick_Mach " : Inport  Port=2  PortWidth=-1  SampleTime=-1  DataType=auto
      settings: SignalType=auto
  "FCS_lat_stick_Altitude " : Inport  Port=3  PortWidth=-1  SampleTime=-1  DataType=auto
      settings: SignalType=auto
  Degrees to Radians : simulink_extras/Transformations/Degrees to Radians
  Gain : Gain  Gain=180/80  SaturateOnIntegerOverflow=on
  Saturation : Saturate  UpperLimit=80  LowerLimit=-80
  Terminator : Terminator
  Terminator 2 : Terminator
  FCS_lat_stick_p : Outport  Port=1
  wires:
  "FCS_lat_stick_Fas "/1 -> Saturation/1
  Degrees to Radians/1 -> FCS_lat_stick_p/1
  Saturation/1 -> Gain/1
  Gain/1 -> Degrees to Radians/1
  "FCS_lat_stick_Mach "/1 -> Terminator/1
  "FCS_lat_stick_Altitude "/1 -> Terminator 2/1

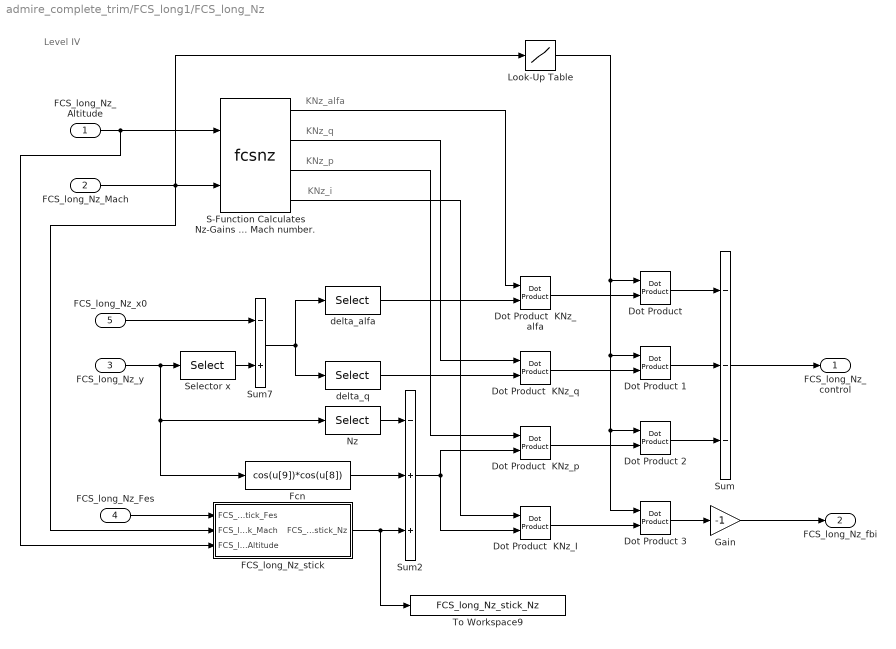
== system admire_complete_trim/FCS_long1/FCS_long_Nz ==
  note: KNz_alfa
  note: KNz_q
  note: KNz_p
  note: KNz_i
  note: Level IV
  "FCS_long_Nz_Altitude " : Inport  Port=1  PortWidth=-1  SampleTime=-1  DataType=auto
      settings: SignalType=auto
  "FCS_long_Nz_Mach " : Inport  Port=2  PortWidth=-1  SampleTime=-1  DataType=auto
      settings: SignalType=auto
  FCS_long_Nz_y : Inport  Port=3  PortWidth=-1  SampleTime=-1  DataType=auto
      settings: SignalType=auto
  FCS_long_Nz_Fes : Inport  Port=4  PortWidth=-1  SampleTime=-1  DataType=auto
      settings: SignalType=auto
  FCS_long_Nz_x0 : Inport  Port=5  PortWidth=-1  SampleTime=-1  DataType=auto
      settings: SignalType=auto
  Dot Product {,1..3} (4 alike) : simulink3/Math/Dot Product
  Dot Product  KNz_I : simulink3/Math/Dot Product
  Dot Product  KNz_alfa : simulink3/Math/Dot Product
  Dot Product  KNz_p : simulink3/Math/Dot Product
  Dot Product  KNz_q : simulink3/Math/Dot Product
  FCS_long_Nz_stick : Subsystem
      mask Display: disp('FCS_long_Nz_stick')
  Fcn : Fcn  Expr=cos(u[9])*cos(u[8])
  Gain : Gain  Gain=-1  SaturateOnIntegerOverflow=on
  Look-Up Table : Lookup  InputValues=[0 0.58 0.62 2.5]  OutputValues=[0 0 1 1]
  Nz : Selector  Elements=19  InputPortWidth=28
  S-Function Calculates Nz-Gains as a function of altitude and Mach number. : S-Function  FunctionName=fcsnz  PortCounts=[]  SFunctionModules=''
  Selector x : Selector  Elements=[1:12]  InputPortWidth=28
  Sum : Sum  Inputs=---  SaturateOnIntegerOverflow=on
  Sum2 : Sum  Inputs=-++  SaturateOnIntegerOverflow=on
  Sum7 : Sum  Inputs=-+  SaturateOnIntegerOverflow=on
  To Workspace9 : ToWorkspace  VariableName=FCS_long_Nz_stick_Nz  SampleTime=-1  SaveFormat=Matrix
  delta_alfa : Selector  Elements=2  InputPortWidth=12
  delta_q : Selector  Elements=5  InputPortWidth=12
  FCS_long_Nz_control : Outport  Port=1
  FCS_long_Nz_fbi : Outport  Port=2
  wires:
  Nz/1 -> Sum2/1
  FCS_long_Nz_Fes/1 -> FCS_long_Nz_stick/1("FCS_long_Nz_stick_Fes ")
  Selector x/1 -> Sum7/2
  FCS_long_Nz_x0/1 -> Sum7/1
  Sum7/1 -> delta_alfa/1, delta_q/1
  FCS_long_Nz_y/1 -> Selector x/1, Nz/1, Fcn/1
  "FCS_long_Nz_Mach "/1 -> S-Function Calculates Nz-Gains as a function of altitude and Mach number./2, Look-Up Table/1, FCS_long_Nz_stick/2(FCS_long_Nz_stick_Mach)
  Sum2/1 -> Dot Product  KNz_p/2, Dot Product  KNz_I/2
  S-Function Calculates Nz-Gains as a function of altitude and Mach number./4 -> Dot Product  KNz_I/1
  delta_alfa/1 -> Dot Product  KNz_alfa/2
  delta_q/1 -> Dot Product  KNz_q/2
  S-Function Calculates Nz-Gains as a function of altitude and Mach number./3 -> Dot Product  KNz_p/1
  S-Function Calculates Nz-Gains as a function of altitude and Mach number./2 -> Dot Product  KNz_q/1
  S-Function Calculates Nz-Gains as a function of altitude and Mach number./1 -> Dot Product  KNz_alfa/1
  "Dot Product "/1 -> Sum/1
  Dot Product  KNz_alfa/1 -> "Dot Product "/2
  Dot Product 1/1 -> Sum/2
  Dot Product  KNz_q/1 -> Dot Product 1/2
  Look-Up Table/1 -> "Dot Product "/1, Dot Product 1/1, Dot Product 2/1, Dot Product 3/1
  Dot Product 2/1 -> Sum/3
  Dot Product  KNz_p/1 -> Dot Product 2/2
  Dot Product  KNz_I/1 -> Dot Product 3/2
  Sum/1 -> FCS_long_Nz_control/1
  Gain/1 -> FCS_long_Nz_fbi/1
  Dot Product 3/1 -> Gain/1
  "FCS_long_Nz_Altitude "/1 -> S-Function Calculates Nz-Gains as a function of altitude and Mach number./1, FCS_long_Nz_stick/3("FCS_long_Nz_stick_Altitude ")
  FCS_long_Nz_stick/1(FCS_long_Nz_stick_Nz) -> To Workspace9/1, Sum2/3
  Fcn/1 -> Sum2/2

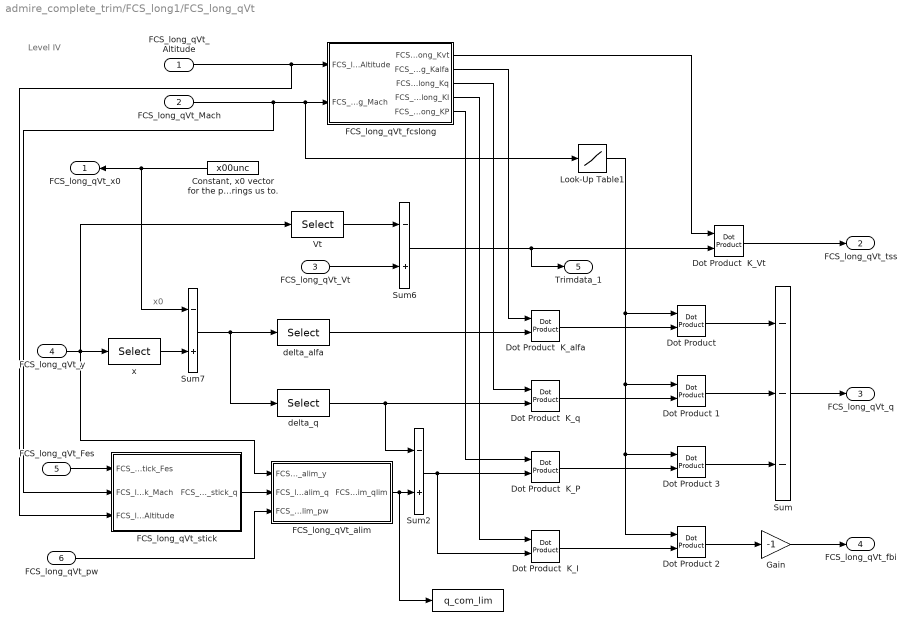
== system admire_complete_trim/FCS_long1/FCS_long_qVt ==
  note: x0
  note: Level IV
  FCS_long_qVt_Altitude : Inport  Port=1  PortWidth=-1  SampleTime=-1  DataType=auto
      settings: SignalType=auto
  FCS_long_qVt_Mach : Inport  Port=2  PortWidth=-1  SampleTime=-1  DataType=auto
      settings: SignalType=auto
  FCS_long_qVt_Vt : Inport  Port=3  PortWidth=-1  SampleTime=-1  DataType=auto
      settings: SignalType=auto
  FCS_long_qVt_y : Inport  Port=4  PortWidth=-1  SampleTime=-1  DataType=auto
      settings: SignalType=auto
  FCS_long_qVt_Fes : Inport  Port=5  PortWidth=-1  SampleTime=-1  DataType=auto
      settings: SignalType=auto
  "FCS_long_qVt_pw " : Inport  Port=6  PortWidth=-1  SampleTime=-1  DataType=auto
      settings: SignalType=auto
  " " : ToWorkspace  VariableName=q_com_lim  SampleTime=-1  SaveFormat=Matrix
  "Constant, x0 vector for the point that the sensor uncertainties  brings us to." : Constant  Orientation=left  Value=x00unc
  Dot Product {,1..3} (4 alike) : simulink3/Math/Dot Product
  Dot Product  K_I : simulink3/Math/Dot Product
  Dot Product  K_P : simulink3/Math/Dot Product
  Dot Product  K_Vt : simulink3/Math/Dot Product
  Dot Product  K_alfa : simulink3/Math/Dot Product
  Dot Product  K_q : simulink3/Math/Dot Product
  FCS_long_qVt_alim : Subsystem
      mask Display: disp('FCS_long_qVt_alim')
  FCS_long_qVt_fcslong : Subsystem
      mask Display: disp('FCS_long_qVt_fcslong')
  FCS_long_qVt_stick : Subsystem
      mask Display: disp('FCS_long_qVt_stick')
  Gain : Gain  Gain=-1  SaturateOnIntegerOverflow=on
  Look-Up Table1 : Lookup  InputValues=[0 0.58 0.62 2.5]  OutputValues=[1 1 0 0]
  Sum : Sum  Inputs=---  SaturateOnIntegerOverflow=on
  Sum2 : Sum  Inputs=-+  SaturateOnIntegerOverflow=on
  Sum6 : Sum  Inputs=-+  SaturateOnIntegerOverflow=on
  Sum7 : Sum  Inputs=-+  SaturateOnIntegerOverflow=on
  Vt : Selector  Elements=1  InputPortWidth=28
  delta_alfa : Selector  Elements=2  InputPortWidth=12
  delta_q : Selector  Elements=5  InputPortWidth=12
  x : Selector  Elements=[1:12]  InputPortWidth=28
  FCS_long_qVt_x0 : Outport  Orientation=left  Port=1
  FCS_long_qVt_tss : Outport  Port=2
  FCS_long_qVt_q : Outport  Port=3
  FCS_long_qVt_fbi : Outport  Port=4
  Trimdata_1 : Outport  Port=5
  wires:
  FCS_long_qVt_fcslong/4(FCS_long_qVt_fcslong_KI) -> Dot Product  K_I/1
  FCS_long_qVt_fcslong/5(FCS_long_qVt_fcslong_KP) -> Dot Product  K_P/1
  FCS_long_qVt_Altitude/1 -> FCS_long_qVt_fcslong/1(FCS_long_qVt_fcslong_Altitude), FCS_long_qVt_stick/3("FCS_long_qVt_stick_Altitude ")
  FCS_long_qVt_Mach/1 -> FCS_long_qVt_fcslong/2(FCS_long_qVt_fcslong_Mach), Look-Up Table1/1, FCS_long_qVt_stick/2("FCS_long_qVt_stick_Mach ")
  delta_alfa/1 -> Dot Product  K_alfa/2
  x/1 -> Sum7/2
  Sum7/1 -> delta_alfa/1, delta_q/1
  delta_q/1 -> Dot Product  K_q/2, Sum2/1
  FCS_long_qVt_y/1 -> x/1, Vt/1, FCS_long_qVt_alim/1(FCS_long_qVt_alim_y)
  FCS_long_qVt_Fes/1 -> FCS_long_qVt_stick/1("FCS_long_qVt_stick_Fes ")
  FCS_long_qVt_alim/1(FCS_long_qVt_alim_qlim) -> Sum2/2, " "/1
  FCS_long_qVt_stick/1("FCS_long_qVt_stick_q ") -> FCS_long_qVt_alim/2("FCS_long_qVt_alim_q ")
  "FCS_long_qVt_pw "/1 -> FCS_long_qVt_alim/3(FCS_long_qVt_alim_pw)
  Dot Product  K_Vt/1 -> FCS_long_qVt_tss/1
  FCS_long_qVt_fcslong/1(FCS_long_qVt_fcslong_Kvt) -> Dot Product  K_Vt/1
  Sum2/1 -> Dot Product  K_P/2, Dot Product  K_I/2
  Dot Product  K_P/1 -> Dot Product 3/2
  Dot Product  K_I/1 -> Dot Product 2/2
  Sum/1 -> FCS_long_qVt_q/1
  Dot Product  K_q/1 -> Dot Product 1/2
  Dot Product 1/1 -> Sum/2
  "Dot Product "/1 -> Sum/1
  Dot Product  K_alfa/1 -> "Dot Product "/2
  Look-Up Table1/1 -> "Dot Product "/1, Dot Product 1/1, Dot Product 2/1, Dot Product 3/1
  Dot Product 3/1 -> Sum/3
  Gain/1 -> FCS_long_qVt_fbi/1
  Dot Product 2/1 -> Gain/1
  FCS_long_qVt_fcslong/3(FCS_long_qVt_fcslong_Kq) -> Dot Product  K_q/1
  FCS_long_qVt_fcslong/2(FCS_long_qVt_fcslong_Kalfa) -> Dot Product  K_alfa/1
  FCS_long_qVt_Vt/1 -> Sum6/2
  Sum6/1 -> Dot Product  K_Vt/2, Trimdata_1/1
  Vt/1 -> Sum6/1
  "Constant, x0 vector for the point that the sensor uncertainties  brings us to."/1 -> FCS_long_qVt_x0/1, Sum7/1

== system admire_complete_trim/Sensor models/Subsystem To Gain-Scheduling ==
  note: Level III
  Vt [m/s] : Inport  Port=1  PortWidth=-1  SampleTime=-1  DataType=auto
      settings: SignalType=auto
  alt [m] : Inport  Port=2  PortWidth=-1  SampleTime=-1  DataType=auto
      settings: SignalType=auto
  S-Function : S-Function  FunctionName=machno  PortCounts=[]  SFunctionModules=''
  Mach : Outport  Port=1
  wires:
  Vt [m/s]/1 -> S-Function/1
  S-Function/1 -> Mach/1
  alt [m]/1 -> S-Function/2

== system admire_complete_trim/FCS_long1/FCS_long_Nz/FCS_long_Nz_stick ==
  note: Level V
  "FCS_long_Nz_stick_Fes " : Inport  Port=1  PortWidth=-1  SampleTime=-1  DataType=auto
      settings: SignalType=auto
  FCS_long_Nz_stick_Mach : Inport  Port=2  PortWidth=-1  SampleTime=-1  DataType=auto
      settings: SignalType=auto
  "FCS_long_Nz_stick_Altitude " : Inport  Port=3  PortWidth=-1  SampleTime=-1  DataType=auto
      settings: SignalType=auto
  Gain : Gain  Gain=8/80  SaturateOnIntegerOverflow=on
  Saturation [-40,+80]   [Newton] : Saturate  UpperLimit=80  LowerLimit=-40
  Terminator : Terminator
  Terminator 2 : Terminator
  FCS_long_Nz_stick_Nz : Outport  Port=1
  wires:
  "FCS_long_Nz_stick_Fes "/1 -> Saturation [-40,+80]   [Newton]/1
  Saturation [-40,+80]   [Newton]/1 -> Gain/1
  Gain/1 -> FCS_long_Nz_stick_Nz/1
  "FCS_long_Nz_stick_Altitude "/1 -> Terminator 2/1
  FCS_long_Nz_stick_Mach/1 -> Terminator/1

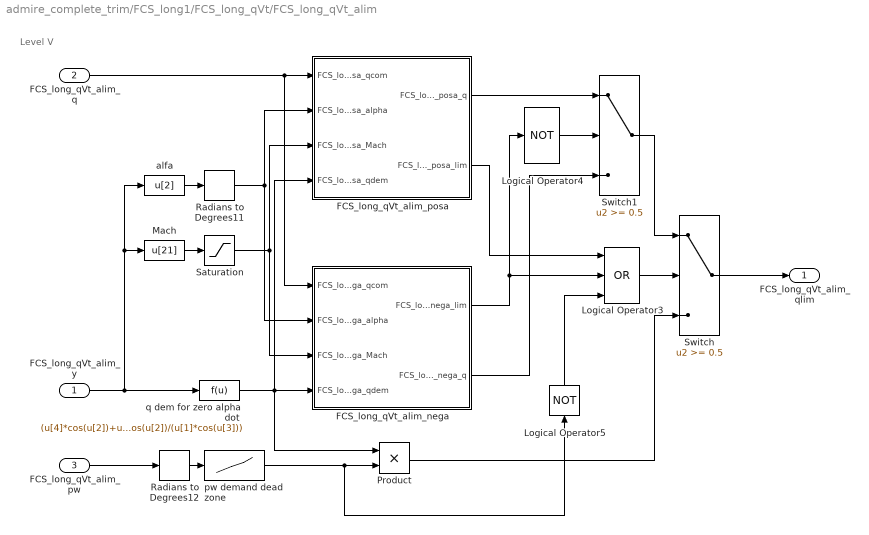
== system admire_complete_trim/FCS_long1/FCS_long_qVt/FCS_long_qVt_alim ==
  note: Level V
  FCS_long_qVt_alim_y : Inport  Port=1  PortWidth=-1  SampleTime=-1  DataType=auto
      settings: SignalType=auto
  "FCS_long_qVt_alim_q " : Inport  Port=2  PortWidth=-1  SampleTime=-1  DataType=auto
      settings: SignalType=auto
  FCS_long_qVt_alim_pw : Inport  Port=3  PortWidth=-1  SampleTime=-1  DataType=auto
      settings: SignalType=auto
  FCS_long_qVt_alim_nega : Subsystem
      mask Display: disp('FCS_long_qVt_alim\nnegative alpha')
  FCS_long_qVt_alim_posa : Subsystem
      mask Display: disp('FCS_long_qVt_alim\npositive alpha')
  Logical Operator3 : Logic  Operator=OR  Inputs=3
  Logical Operator4 : Logic  Operator=NOT  Inputs=1
  Logical Operator5 : Logic  Orientation=up  Operator=NOT  Inputs=1
  Mach : Fcn  Expr=u[21]
  Product : Product  Inputs=2  SaturateOnIntegerOverflow=on
  Radians to Degrees11 : simulink_extras/Transformations/Radians to Degrees
  Radians to Degrees12 : simulink_extras/Transformations/Radians to Degrees
  Saturation : Saturate  UpperLimit=2.5  LowerLimit=0
  Switch : Switch  Threshold=0.5
  Switch1 : Switch  Threshold=0.5
  alfa : Fcn  Expr=u[2]
  pw demand dead zone : Lookup  InputValues=[-180 -10 -8 8 10 180]  OutputValues=[0 0 0 0 0 0]
  "q dem for zero alpha dot " : Fcn  Expr=(u[4]*cos(u[2])+u[6]*sin(u[2]))*tan(u[3])+(u[19]-cos(u[8])*cos(u[9]))*9.80665*cos(u[2])/(u[1]*cos(u[3]))
  FCS_long_qVt_alim_qlim : Outport  Port=1
  wires:
  Logical Operator3/1 -> Switch/2
  Switch1/1 -> Switch/1
  alfa/1 -> Radians to Degrees11/1
  Mach/1 -> Saturation/1
  Radians to Degrees11/1 -> FCS_long_qVt_alim_posa/2("FCS_long_qVt_alim_posa_alpha "), FCS_long_qVt_alim_nega/2("FCS_long_qVt_alim_nega_alpha ")
  Saturation/1 -> FCS_long_qVt_alim_posa/3("FCS_long_qVt_alim_posa_Mach "), FCS_long_qVt_alim_nega/3("FCS_long_qVt_alim_nega_Mach ")
  FCS_long_qVt_alim_y/1 -> "q dem for zero alpha dot "/1, Mach/1, alfa/1
  "q dem for zero alpha dot "/1 -> FCS_long_qVt_alim_nega/4("FCS_long_qVt_alim_nega_qdem "), FCS_long_qVt_alim_posa/4("FCS_long_qVt_alim_posa_qdem "), Product/1
  "FCS_long_qVt_alim_q "/1 -> FCS_long_qVt_alim_posa/1("FCS_long_qVt_alim_posa_qcom "), FCS_long_qVt_alim_nega/1("FCS_long_qVt_alim_nega_qcom ")
  FCS_long_qVt_alim_nega/2("FCS_long_qVt_alim_nega_q ") -> Switch1/3
  FCS_long_qVt_alim_posa/1(FCS_long_qVt_alim_posa_q) -> Switch1/1
  Logical Operator4/1 -> Switch1/2
  FCS_long_qVt_alim_nega/1(FCS_long_qVt_alim_nega_lim) -> Logical Operator4/1, Logical Operator3/2
  FCS_long_qVt_alim_posa/2(FCS_long_qVt_alim_posa_lim) -> Logical Operator3/1
  Switch/1 -> FCS_long_qVt_alim_qlim/1
  Radians to Degrees12/1 -> pw demand dead zone/1
  Product/1 -> Switch/3
  FCS_long_qVt_alim_pw/1 -> Radians to Degrees12/1
  pw demand dead zone/1 -> Product/2, Logical Operator5/1
  Logical Operator5/1 -> Logical Operator3/3

== system admire_complete_trim/FCS_long1/FCS_long_qVt/FCS_long_qVt_fcslong ==
  note: Level V
  note: S-function
  FCS_long_qVt_fcslong_Altitude : Inport  Port=1  PortWidth=-1  SampleTime=-1  DataType=auto
      settings: SignalType=auto
  FCS_long_qVt_fcslong_Mach : Inport  Port=2  PortWidth=-1  SampleTime=-1  DataType=auto
      settings: SignalType=auto
  S-Function1 : S-Function  FunctionName=fcslongitudinal  PortCounts=[]  SFunctionModules=''
  FCS_long_qVt_fcslong_Kvt : Outport  Port=1
  FCS_long_qVt_fcslong_Kalfa : Outport  Port=2
  FCS_long_qVt_fcslong_Kq : Outport  Port=3
  FCS_long_qVt_fcslong_KI : Outport  Port=4
  FCS_long_qVt_fcslong_KP : Outport  Port=5
  wires:
  FCS_long_qVt_fcslong_Mach/1 -> S-Function1/2
  FCS_long_qVt_fcslong_Altitude/1 -> S-Function1/1
  S-Function1/1 -> FCS_long_qVt_fcslong_Kalfa/1
  S-Function1/2 -> FCS_long_qVt_fcslong_KI/1
  S-Function1/3 -> FCS_long_qVt_fcslong_KP/1
  S-Function1/4 -> FCS_long_qVt_fcslong_Kq/1
  S-Function1/5 -> FCS_long_qVt_fcslong_Kvt/1
